simulink model "NN_v01"  (R2018b)
settings: Solver=VariableStepAuto  StartTime=0.0  StopTime=10.0  RelTol=1e-3
values from neighbouring files (symbols this model uses):
  B = 0.5    [Matlab_Newton_simulation_v01.m]    (also in NewtonMethod.m; NewtonMethod_2.m = 0.3; System_parameters.m = 0.3)
  b = f    (= 0.01)    [Matlab_Newton_simulation_v01.m]    (also in NewtonMethod.m; System_parameters.m)
  in_NN_data = [0 -100 -100 -100 -100 -100 -100 -100 -100 -100 -100 -100 ... (160801 elements, 401x401)]    [NN_IO_data.mat]    (also in NN_generate_input_data.m = con2seq(in_NN_data); NN_modelling_v02.m = con2seq(in_NN_data); NN_modelling_v03.m = con2seq(in_NN_data))
  l = 0.1    [Matlab_Newton_simulation_v01.m]    (also in NewtonMethod.m; NewtonMethod_2.m; System_parameters.m)
  m = 0.04    [Matlab_Newton_simulation_v01.m]    (also in NewtonMethod.m = 0.1; NewtonMethod_2.m; System_parameters.m)
  R = 1    [Matlab_Newton_simulation_v01.m]    (also in NewtonMethod.m; NewtonMethod_2.m = 0.1; System_parameters.m = 0.1)
libraries: neural x128
(part 1 of 5)
settings Model: Creator=Tyson  LastModifiedBy=Tyson

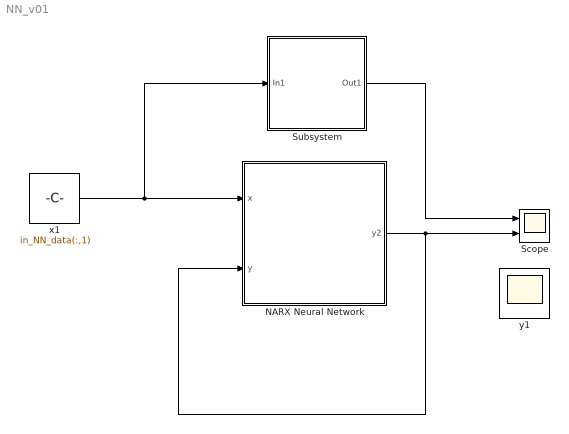
== system NN_v01 ==
  NARX Neural Network : Subsystem  mask{pi_input_1_delayed_1=-1, pi_input_1_delayed_2=-1, pi_input_2_delayed_1=-1, pi_input_2_delayed_2=-1}
      mask prompts: pi_input_1_delayed_1 "Preprocessed initial input 1 state at timestep 0."; pi_input_1_delayed_2 "Preprocessed initial input 1 state at timestep -1."; pi_input_2_delayed_1 "Preprocessed initial input 2 state at timestep 0."; pi_input_2_delayed_2 "Preprocessed initial input 2 state at timestep -1."
      mask help: NARX Neural Network
      mask Display: e = 0.06;c1 = [120 150 230]/255;c2 = ([120 150 230]+0)/383;c3 = ([120 150 230]+128)/383;patch([0 1 1 0],[0 0 1 1],c1);patch([0 1 1 1-e 1-e 0+e],[0 0 1 1-e 0+e 0+e],c2);patch([0 0 1 1-e 0+e 0+e],[0 1 1 1-e 1-e 0+e],c3);plot([0 1 1 0 0],[0 0 1 1 0]);fprintf('NNET');port_label('input',1,' x');port_label('input',2,' y');port_label('output',1,'y2 ');
  Scope : Scope  NumInputPorts=2
  Subsystem : Subsystem
      mask DialogControl Control2 Prompt: BlackBox
  x1 : Constant  Value=in_NN_data(:,1)  SampleTime=-1
      mask Display: e = 0.06;c1 = [120 230 180]/255;c2 = ([120 230 180]+0)/(256+128);c3 = ([120 230 180]+128)/(256+128);patch([0 1 1 0],[0 0 1 1],c1);patch([0 1 1 1-e 1-e 0+e],[0 0 1 1-e 0+e 0+e],c2);patch([0 0 1 1-e 0+e 0+e],[0 1 1 1-e 1-e 0+e],c3);plot([0 1 1 0 0],[0 0 1 1 0]);disp('Constant');
  y1 : Scope
      mask Display: e = 0.06;c1 = [120 230 180]/255;c2 = ([120 230 180]+0)/(256+128);c3 = ([120 230 180]+128)/(256+128);patch([0 1 1 0],[0 0 1 1],c1);patch([0 1 1 1-e 1-e 0+e],[0 0 1 1-e 0+e 0+e],c2);patch([0 0 1 1-e 0+e 0+e],[0 1 1 1-e 1-e 0+e],c3);plot([0 1 1 0 0],[0 0 1 1 0]);plot([0.15 0.85 0.85 0.15 0.15],[0.5 0.5 0.85 0.85 0.5]);
  wires:
  x1/1 -> Subsystem/1(In1), NARX Neural Network/1(x)
  NARX Neural Network/1(y2) -> NARX Neural Network/2(y), Scope/2
  Subsystem/1(Out1) -> Scope/1

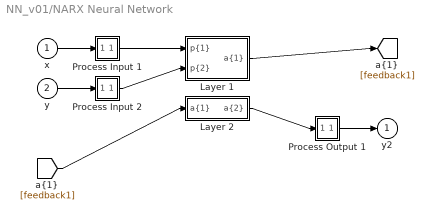
== system NN_v01/NARX Neural Network ==
  x : Inport  PortDimensions=101  SampleTime=1
      mask Display: e = 0.06;c1 = [120 230 180]/255;c2 = ([120 230 180]+0)/(256+128);c3 = ([120 230 180]+128)/(256+128);patch([0 1 1 0],[0 0 1 1],c1);patch([0 1 1 1-e 1-e 0+e],[0 0 1 1-e 0+e 0+e],c2);patch([0 0 1 1-e 0+e 0+e],[0 1 1 1-e 1-e 0+e],c3);plot([0 1 1 0 0],[0 0 1 1 0]);
  y : Inport  Port=2  PortDimensions=101  SampleTime=1
      mask Display: e = 0.06;c1 = [120 230 180]/255;c2 = ([120 230 180]+0)/(256+128);c3 = ([120 230 180]+128)/(256+128);patch([0 1 1 0],[0 0 1 1],c1);patch([0 1 1 1-e 1-e 0+e],[0 0 1 1-e 0+e 0+e],c2);patch([0 0 1 1-e 0+e 0+e],[0 1 1 1-e 1-e 0+e],c3);plot([0 1 1 0 0],[0 0 1 1 0]);
  Layer 1 : Subsystem
      mask Display: e = 0.06;c1 = [120 150 230]/255;c2 = ([120 150 230]+0)/383;c3 = ([120 150 230]+128)/383;patch([0 1 1 0],[0 0 1 1],c1);patch([0 1 1 1-e 1-e 0+e],[0 0 1 1-e 0+e 0+e],c2);patch([0 0 1 1-e 0+e 0+e],[0 1 1 1-e 1-e 0+e],c3);plot([0 1 1 0 0],[0 0 1 1 0]);
  Layer 2 : Subsystem
      mask Display: e = 0.06;c1 = [120 150 230]/255;c2 = ([120 150 230]+0)/383;c3 = ([120 150 230]+128)/383;patch([0 1 1 0],[0 0 1 1],c1);patch([0 1 1 1-e 1-e 0+e],[0 0 1 1-e 0+e 0+e],c2);patch([0 0 1 1-e 0+e 0+e],[0 1 1 1-e 1-e 0+e],c3);plot([0 1 1 0 0],[0 0 1 1 0]);
  Process Input 1 : Subsystem
      mask Display: e = 0.06;c1 = [120 150 230]/255;c2 = ([120 150 230]+0)/383;c3 = ([120 150 230]+128)/383;patch([0 1 1 0],[0 0 1 1],c1);patch([0 1 1 1-e 1-e 0+e],[0 0 1 1-e 0+e 0+e],c2);patch([0 0 1 1-e 0+e 0+e],[0 1 1 1-e 1-e 0+e],c3);plot([0 1 1 0 0],[0 0 1 1 0]);
  Process Input 2 : Subsystem
      mask Display: e = 0.06;c1 = [120 150 230]/255;c2 = ([120 150 230]+0)/383;c3 = ([120 150 230]+128)/383;patch([0 1 1 0],[0 0 1 1],c1);patch([0 1 1 1-e 1-e 0+e],[0 0 1 1-e 0+e 0+e],c2);patch([0 0 1 1-e 0+e 0+e],[0 1 1 1-e 1-e 0+e],c3);plot([0 1 1 0 0],[0 0 1 1 0]);
  Process Output 1 : Subsystem
      mask Display: e = 0.06;c1 = [120 150 230]/255;c2 = ([120 150 230]+0)/383;c3 = ([120 150 230]+128)/383;patch([0 1 1 0],[0 0 1 1],c1);patch([0 1 1 1-e 1-e 0+e],[0 0 1 1-e 0+e 0+e],c2);patch([0 0 1 1-e 0+e 0+e],[0 1 1 1-e 1-e 0+e],c3);plot([0 1 1 0 0],[0 0 1 1 0]);
  y2 : Outport  InitialOutput=[0;0;0;0;0;0;0;0;0;0;0;0;0;0;0;0;0;0;0;0;0;0;0;0;0;0;0;0;0;0;0;0;0;0;0;0;0;0;0;0;0;0;0;0;0;0;0;0;0;0;0;0;0;0;0;0;0;0;0;0;0;0;0;0;0;0;0;0;0;0;0;0;0;0;0;0;0;0;0;0;0;0;0;0;0;0;0;0;0;0;0;0;0;0;0;0;0;0;0;0;0]
      mask Display: e = 0.06;c1 = [120 230 180]/255;c2 = ([120 230 180]+0)/(256+128);c3 = ([120 230 180]+128)/(256+128);patch([0 1 1 0],[0 0 1 1],c1);patch([0 1 1 1-e 1-e 0+e],[0 0 1 1-e 0+e 0+e],c2);patch([0 0 1 1-e 0+e 0+e],[0 1 1 1-e 1-e 0+e],c3);plot([0 1 1 0 0],[0 0 1 1 0]);
  wires:
  x/1 -> Process Input 1/1(x)
  y/1 -> Process Input 2/1(x)
  Process Output 1/1(y) -> y2/1
  Process Input 1/1(p) -> Layer 1/1("p{1}")
  Process Input 2/1(p) -> Layer 1/2("p{2}")
  Layer 1/1("a{1}") -> [feedback1]
  [feedback1] -> Layer 2/1("a{1} ")
  Layer 2/1("a{2}") -> Process Output 1/1(a)

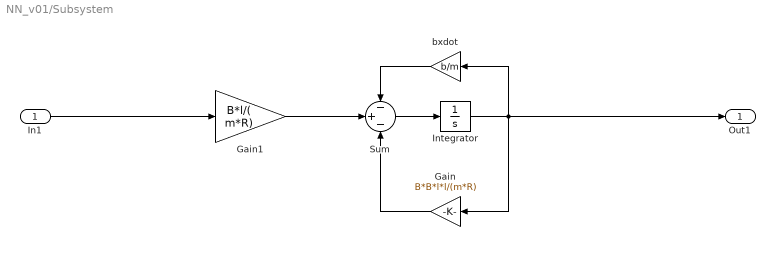
== system NN_v01/Subsystem ==
  In1 : Inport
  Gain : Gain  Gain=B*B*l*l/(m*R)
  Gain1 : Gain  Gain=B*l/( m*R)
  Integrator : Integrator
  Sum : Sum  Inputs=-+-
  bxdot : Gain  Gain=b/m
  Out1 : Outport
  wires:
  Sum/1 -> Integrator/1
  Gain/1 -> Sum/3
  Gain1/1 -> Sum/2
  bxdot/1 -> Sum/1
  Integrator/1 -> Out1/1, bxdot/1, Gain/1
  In1/1 -> Gain1/1

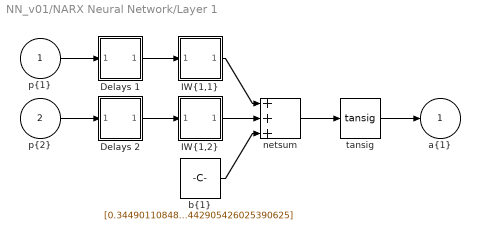
== system NN_v01/NARX Neural Network/Layer 1 ==
  "p{1}" : Inport  PortDimensions=100  SampleTime=1
      mask Display: e = 0.06;c1 = [120 230 180]/255;c2 = ([120 230 180]+0)/(256+128);c3 = ([120 230 180]+128)/(256+128);patch([0 1 1 0],[0 0 1 1],c1);patch([0 1 1 1-e 1-e 0+e],[0 0 1 1-e 0+e 0+e],c2);patch([0 0 1 1-e 0+e 0+e],[0 1 1 1-e 1-e 0+e],c3);plot([0 1 1 0 0],[0 0 1 1 0]);
  "p{2}" : Inport  Port=2  PortDimensions=100  SampleTime=1
      mask Display: e = 0.06;c1 = [120 230 180]/255;c2 = ([120 230 180]+0)/(256+128);c3 = ([120 230 180]+128)/(256+128);patch([0 1 1 0],[0 0 1 1],c1);patch([0 1 1 1-e 1-e 0+e],[0 0 1 1-e 0+e 0+e],c2);patch([0 0 1 1-e 0+e 0+e],[0 1 1 1-e 1-e 0+e],c3);plot([0 1 1 0 0],[0 0 1 1 0]);
  Delays 1 : Subsystem
      mask Display: e = 0.06;c1 = [120 150 230]/255;c2 = ([120 150 230]+0)/383;c3 = ([120 150 230]+128)/383;patch([0 1 1 0],[0 0 1 1],c1);patch([0 1 1 1-e 1-e 0+e],[0 0 1 1-e 0+e 0+e],c2);patch([0 0 1 1-e 0+e 0+e],[0 1 1 1-e 1-e 0+e],c3);plot([0 1 1 0 0],[0 0 1 1 0]);disp('1-2');
  Delays 2 : Subsystem
      mask Display: e = 0.06;c1 = [120 150 230]/255;c2 = ([120 150 230]+0)/383;c3 = ([120 150 230]+128)/383;patch([0 1 1 0],[0 0 1 1],c1);patch([0 1 1 1-e 1-e 0+e],[0 0 1 1-e 0+e 0+e],c2);patch([0 0 1 1-e 0+e 0+e],[0 1 1 1-e 1-e 0+e],c3);plot([0 1 1 0 0],[0 0 1 1 0]);disp('1-2');
  "IW{1,1}" : Subsystem
      mask Display: e = 0.06;c1 = [120 150 230]/255;c2 = ([120 150 230]+0)/383;c3 = ([120 150 230]+128)/383;patch([0 1 1 0],[0 0 1 1],c1);patch([0 1 1 1-e 1-e 0+e],[0 0 1 1-e 0+e 0+e],c2);patch([0 0 1 1-e 0+e 0+e],[0 1 1 1-e 1-e 0+e],c3);plot([0 1 1 0 0],[0 0 1 1 0]);disp('W');
  "IW{1,2}" : Subsystem
      mask Display: e = 0.06;c1 = [120 150 230]/255;c2 = ([120 150 230]+0)/383;c3 = ([120 150 230]+128)/383;patch([0 1 1 0],[0 0 1 1],c1);patch([0 1 1 1-e 1-e 0+e],[0 0 1 1-e 0+e 0+e],c2);patch([0 0 1 1-e 0+e 0+e],[0 1 1 1-e 1-e 0+e],c3);plot([0 1 1 0 0],[0 0 1 1 0]);disp('W');
  "b{1}" : Constant  Value=[0.34490110848554278444311194107285700738430023193359375;-0.55926377926860249001350666731013916432857513427734375;0.08828364470528819729633340784857864491641521453857421875;0.47063354920653821533704785906593315303325653076171875;0.0163244137557161834994889915151361492462456226348876953125;0.380666321851039490820056698794360272586345672607421875;0.473534513113422317331924205063842236995697021484375;0.0303941138129983599858174869723370647989213466644287109375;-0.00010565009611801054359263296600346393461222760379314422607421875;-0.0342241349195050725828792792526655830442905426025390625]
      mask Display: e = 0.06;c1 = [120 150 230]/255;c2 = ([120 150 230]+0)/383;c3 = ([120 150 230]+128)/383;patch([0 1 1 0],[0 0 1 1],c1);patch([0 1 1 1-e 1-e 0+e],[0 0 1 1-e 0+e 0+e],c2);patch([0 0 1 1-e 0+e 0+e],[0 1 1 1-e 1-e 0+e],c3);plot([0 1 1 0 0],[0 0 1 1 0]);disp('b');
  netsum : Sum  Inputs=3  SaturateOnIntegerOverflow=on  InputSameDT=on  OutDataTypeStr=Inherit: Same as first input
      mask Display: e = 0.06;c1 = [120 150 230]/255;c2 = ([120 150 230]+0)/383;c3 = ([120 150 230]+128)/383;patch([0 1 1 0],[0 0 1 1],c1);patch([0 1 1 1-e 1-e 0+e],[0 0 1 1-e 0+e 0+e],c2);patch([0 0 1 1-e 0+e 0+e],[0 1 1 1-e 1-e 0+e],c3);plot([0 1 1 0 0],[0 0 1 1 0]);disp('+');
  tansig : neural/Transfer Functions/tansig
  "a{1}" : Outport  InitialOutput=[0;0;0;0;0;0;0;0;0;0]
      mask Display: e = 0.06;c1 = [120 230 180]/255;c2 = ([120 230 180]+0)/(256+128);c3 = ([120 230 180]+128)/(256+128);patch([0 1 1 0],[0 0 1 1],c1);patch([0 1 1 1-e 1-e 0+e],[0 0 1 1-e 0+e 0+e],c2);patch([0 0 1 1-e 0+e 0+e],[0 1 1 1-e 1-e 0+e],c3);plot([0 1 1 0 0],[0 0 1 1 0]);
  wires:
  "p{1}"/1 -> Delays 1/1("p{1}")
  Delays 1/1("pd{1,1}") -> "IW{1,1}"/1("pd{1,1}")
  "IW{1,1}"/1("iz{1,1}") -> netsum/1
  "p{2}"/1 -> Delays 2/1("p{1}")
  Delays 2/1("pd{1,2}") -> "IW{1,2}"/1("pd{1,2}")
  "IW{1,2}"/1("iz{1,2}") -> netsum/2
  "b{1}"/1 -> netsum/3
  netsum/1 -> tansig/1
  tansig/1 -> "a{1}"/1

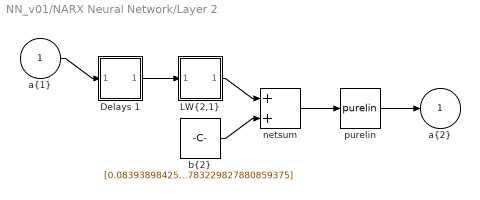
== system NN_v01/NARX Neural Network/Layer 2 ==
  "a{1} " : Inport  PortDimensions=10  SampleTime=1
      mask Display: e = 0.06;c1 = [120 230 180]/255;c2 = ([120 230 180]+0)/(256+128);c3 = ([120 230 180]+128)/(256+128);patch([0 1 1 0],[0 0 1 1],c1);patch([0 1 1 1-e 1-e 0+e],[0 0 1 1-e 0+e 0+e],c2);patch([0 0 1 1-e 0+e 0+e],[0 1 1 1-e 1-e 0+e],c3);plot([0 1 1 0 0],[0 0 1 1 0]);
  Delays 1 : Subsystem
      mask Display: e = 0.06;c1 = [120 150 230]/255;c2 = ([120 150 230]+0)/383;c3 = ([120 150 230]+128)/383;patch([0 1 1 0],[0 0 1 1],c1);patch([0 1 1 1-e 1-e 0+e],[0 0 1 1-e 0+e 0+e],c2);patch([0 0 1 1-e 0+e 0+e],[0 1 1 1-e 1-e 0+e],c3);plot([0 1 1 0 0],[0 0 1 1 0]);disp('0');
  "LW{2,1}" : Subsystem
      mask Display: e = 0.06;c1 = [120 150 230]/255;c2 = ([120 150 230]+0)/383;c3 = ([120 150 230]+128)/383;patch([0 1 1 0],[0 0 1 1],c1);patch([0 1 1 1-e 1-e 0+e],[0 0 1 1-e 0+e 0+e],c2);patch([0 0 1 1-e 0+e 0+e],[0 1 1 1-e 1-e 0+e],c3);plot([0 1 1 0 0],[0 0 1 1 0]);disp('W');
  "b{2}" : Constant  Value=[0.08393898425384989370190425006512668915092945098876953125;0.04747955954920869692248430737890885211527347564697265625;0.02259412956298940955424114918059785850346088409423828125;0.0189850525832074117082992614768954808823764324188232421875;-0.021115224393390634449740872469192254357039928436279296875;-0.0258363266266243007951430854518548585474491119384765625;-0.032480391177460994633907631623515044339001178741455078125;-0.00530185149898763398434997640151777886785566806793212890625;0.00082595733270498269788795209223053461755625903606414794921875;0.00153775931011657248335955383566897580749355256557464599609375;-0.020679742413263597911043945032361079938709735870361328125;-0.0177142011664902405965182907721100491471588611602783203125;-0.032660583320958509745413067548724939115345478057861328125;-0.03167603138593400036171487954561598598957061767578125;-0.02560287967276560217033676281062071211636066436767578125;-0.01468973685666209900990697434508547303266823291778564453125;-0.0287572723231526994336348934666602872312068939208984375;-0.01438192548970657937135175785670071491040289402008056640625;-0.01225306330625217966778794931315132998861372470855712890625;-0.009015829424581602025146054302240372635424137115478515625;-0.0224190206360676824726141376231680624186992645263671875;-0.0162041639024568494276135055542908958159387111663818359375;0.00463628568182163254551841902184605714865028858184814453125;-0.017249539041738481959242790253483690321445465087890625;-0.0093907194819392129925272882928766193799674510955810546875;0.00103156476558706466928327927234931848943233489990234375;-0.0149805915005030397535445985113256028853356838226318359375;-0.0117658372520909083880358281248845742084085941314697265625;-0.002292463185382479125273835762754970346577465534210205078125;-0.0115253284335917853542508026976065593771636486053466796875;-0.000676344485529874715756815106715293950401246547698974609375;-0.0211093999094044103281841984198763384483754634857177734375;-0.0033268637067907619840612110095889875083230435848236083984375;-0.0277640599743354289652419453204856836237013339996337890625;0.00410158032873014603836292479854819248430430889129638671875;-0.019817410413248894018867218846935429610311985015869140625;-0.03181619165364106549542810853381524793803691864013671875;-0.005128465510424081059970280449533674982376396656036376953125;-0.0122950128646857233249978236244714935310184955596923828125;-0.0296459773916183007280711336761669372208416461944580078125;-0.02841264500203134757416734146318049170076847076416015625;-0.0288484832263984948552693055034978897310793399810791015625;-0.0316585468321592122808993963190005160868167877197265625;-0.01425623173418808474488539417279753251932561397552490234375;-0.0326474212064222502061028308162349276244640350341796875;-0.026458854464259225214295412342835334129631519317626953125;-0.041621208256695275962133706570966751314699649810791015625;-0.0323289680718874539167018156149424612522125244140625;-0.0148329882382925264117101704641754622571170330047607421875;-0.01090351148061602555572324746435697306878864765167236328125;-0.038850136436738465228746264301662449724972248077392578125;-0.03859829631133258887043524509863345883786678314208984375;-0.006839581773198071500130534872141652158461511135101318359375;-0.0259010284650814902318582966245230636559426784515380859375;-0.03254737113984364216268119207597919739782810211181640625;-0.02189820350106060076189606888874550350010395050048828125;-0.005298122488479149218287833633667105459608137607574462890625;-0.020306466616356773358109677474203635938465595245361328125;-0.03097649086438274135257842090140911750495433807373046875;-0.0365192638172040784372285315839690156280994415283203125;-0.0156068747337300868516241081351836328394711017608642578125;-0.0275454361412660712893352155106185819022357463836669921875;-0.029019398236701375581869655206901370547711849212646484375;-0.030534494348092237892000611054754699580371379852294921875;-0.0122323399612508480760464379955010372214019298553466796875 ...(+2140 chars)]
      mask Display: e = 0.06;c1 = [120 150 230]/255;c2 = ([120 150 230]+0)/383;c3 = ([120 150 230]+128)/383;patch([0 1 1 0],[0 0 1 1],c1);patch([0 1 1 1-e 1-e 0+e],[0 0 1 1-e 0+e 0+e],c2);patch([0 0 1 1-e 0+e 0+e],[0 1 1 1-e 1-e 0+e],c3);plot([0 1 1 0 0],[0 0 1 1 0]);disp('b');
  netsum : Sum  Inputs=2  SaturateOnIntegerOverflow=on  InputSameDT=on  OutDataTypeStr=Inherit: Same as first input
      mask Display: e = 0.06;c1 = [120 150 230]/255;c2 = ([120 150 230]+0)/383;c3 = ([120 150 230]+128)/383;patch([0 1 1 0],[0 0 1 1],c1);patch([0 1 1 1-e 1-e 0+e],[0 0 1 1-e 0+e 0+e],c2);patch([0 0 1 1-e 0+e 0+e],[0 1 1 1-e 1-e 0+e],c3);plot([0 1 1 0 0],[0 0 1 1 0]);disp('+');
  purelin : neural/Transfer Functions/purelin
  "a{2}" : Outport  InitialOutput=[0;0;0;0;0;0;0;0;0;0;0;0;0;0;0;0;0;0;0;0;0;0;0;0;0;0;0;0;0;0;0;0;0;0;0;0;0;0;0;0;0;0;0;0;0;0;0;0;0;0;0;0;0;0;0;0;0;0;0;0;0;0;0;0;0;0;0;0;0;0;0;0;0;0;0;0;0;0;0;0;0;0;0;0;0;0;0;0;0;0;0;0;0;0;0;0;0;0;0;0]
      mask Display: e = 0.06;c1 = [120 230 180]/255;c2 = ([120 230 180]+0)/(256+128);c3 = ([120 230 180]+128)/(256+128);patch([0 1 1 0],[0 0 1 1],c1);patch([0 1 1 1-e 1-e 0+e],[0 0 1 1-e 0+e 0+e],c2);patch([0 0 1 1-e 0+e 0+e],[0 1 1 1-e 1-e 0+e],c3);plot([0 1 1 0 0],[0 0 1 1 0]);
  wires:
  "a{1} "/1 -> Delays 1/1("p{2}")
  Delays 1/1("pd{2,1}") -> "LW{2,1}"/1("ad{2,1}")
  "LW{2,1}"/1("lz{2,1}") -> netsum/1
  "b{2}"/1 -> netsum/2
  netsum/1 -> purelin/1
  purelin/1 -> "a{2}"/1

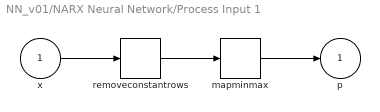
== system NN_v01/NARX Neural Network/Process Input 1 ==
  x : Inport  PortDimensions=101  SampleTime=1
      mask Display: e = 0.06;c1 = [120 230 180]/255;c2 = ([120 230 180]+0)/(256+128);c3 = ([120 230 180]+128)/(256+128);patch([0 1 1 0],[0 0 1 1],c1);patch([0 1 1 1-e 1-e 0+e],[0 0 1 1-e 0+e 0+e],c2);patch([0 0 1 1-e 0+e 0+e],[0 1 1 1-e 1-e 0+e],c3);plot([0 1 1 0 0],[0 0 1 1 0]);
  mapminmax : neural/Processing Functions/mapminmax  xmin=[-50;-50;-50;-50;-50;-50;-50;-50;-50;-50;-50;-50;-50;-50;-50;-50;-50;-50;-50;-50;-50;-50;-50;-50;-50;-50;-50;-50;-50;-50;-50;-50;-50;-50;-50;-50;-50;-50;-50;-50;-50;-50;-50;-50;-50;-50;-50;-50;-50;-50;-50;-50;-50;-50;-50;-50;-50;-50;-50;-50;-50;-50;-50;-50;-50;-50;-50;-50;-50;-50;-50;-50;-50;-50;-50;-50;-50;-50;-50;-50;-50;-50;-50;-50;-50;-50;-50;-50;-50;-50;-50;-50;-50;-50;-50;-50;-50;-50;-50;-50]  xmax=[50;50;50;50;50;50;50;50;50;50;50;50;50;50;50;50;50;50;50;50;50;50;50;50;50;50;50;50;50;50;50;50;50;50;50;50;50;50;50;50;50;50;50;50;50;50;50;50;50;50;50;50;50;50;50;50;50;50;50;50;50;50;50;50;50;50;50;50;50;50;50;50;50;50;50;50;50;50;50;50;50;50;50;50;50;50;50;50;50;50;50;50;50;50;50;50;50;50;50;50]  ymin=-1  ymax=1
  removeconstantrows : neural/Processing Functions/removeconstantrows  inputSize=101  keep=[2 3 4 5 6 7 8 9 10 11 12 13 14 15 16 17 18 19 20 21 22 23 24 25 26 27 28 29 30 31 32 33 34 35 36 37 38 39 40 41 42 43 44 45 46 47 48 49 50 51 52 53 54 55 56 57 58 59 60 61 62 63 64 65 66 67 68 69 70 71 72 73 74 75 76 77 78 79 80 81 82 83 84 85 86 87 88 89 90 91 92 93 94 95 96 97 98 99 100 101]
      settings: SourceProductName=Neural Network Toolbox  SourceProductBaseCode=NN
  p : Outport  PortDimensions=100  SampleTime=1
      mask Display: e = 0.06;c1 = [120 230 180]/255;c2 = ([120 230 180]+0)/(256+128);c3 = ([120 230 180]+128)/(256+128);patch([0 1 1 0],[0 0 1 1],c1);patch([0 1 1 1-e 1-e 0+e],[0 0 1 1-e 0+e 0+e],c2);patch([0 0 1 1-e 0+e 0+e],[0 1 1 1-e 1-e 0+e],c3);plot([0 1 1 0 0],[0 0 1 1 0]);
  wires:
  x/1 -> removeconstantrows/1
  removeconstantrows/1 -> mapminmax/1
  mapminmax/1 -> p/1

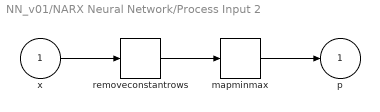
== system NN_v01/NARX Neural Network/Process Input 2 ==
  x : Inport  PortDimensions=101  SampleTime=1
      mask Display: e = 0.06;c1 = [120 230 180]/255;c2 = ([120 230 180]+0)/(256+128);c3 = ([120 230 180]+128)/(256+128);patch([0 1 1 0],[0 0 1 1],c1);patch([0 1 1 1-e 1-e 0+e],[0 0 1 1-e 0+e 0+e],c2);patch([0 0 1 1-e 0+e 0+e],[0 1 1 1-e 1-e 0+e],c3);plot([0 1 1 0 0],[0 0 1 1 0]);
  mapminmax : neural/Processing Functions/mapminmax  xmin=[-18.453125;-54.2205659473063121822633547708;-88.3287647166492035921692149714;-120.854693116249151785268622916;-151.871752252388432680163532495;-181.449938173334970770156360231;-209.655999829087903663094039075;-236.553589703412313838271074928;-262.203407458093295190337812528;-286.663336913571072273043682799;-309.988576675080253153282683343;-332.231764699077018576645059511;-353.443097081062433062470518053;-373.670441332869870620925212279;-392.95944440504888461873633787;-411.353635698119205699185840786;-428.894525295159496636188123375;-445.621697637412523818056797609;-461.572900854303213691309792921;-476.784131949461141175561351702;-491.289718034985355643584625795;-505.122393797273446125473128632;-518.313375369230925571173429489;-530.892430775568186618329491466;-542.88794711015907523687928915;-554.326994597059069747047033161;-565.235387679749578637711238116;-575.637743276468654585187323391;-585.557536333092230051988735795;-595.017152798931306278973352164;-604.037940144996241542685311288;-612.640255538732276363589335233;-620.843511783941039539058692753;-628.666221129561904490401502699;-636.126037046174928946129512042;-643.239794064503257686737924814;-650.023545765817630126548465341;-656.49260100997605604788986966;-662.661558482854275098361540586;-668.544339641130022755532991141;-674.154220128767292408156208694;-679.503859736098547728033736348;-684.605330969112401362508535385;-689.470146293419929861556738615;-694.109284114380670871469192207;-698.533213552016832181834615767;-702.75191806662667204363970086;-706.77491798841094805538887158;-710.611292001956485364644322544;-714.269697634059980373422149569;-717.758390791126998919935431331;-721.085244390236653089232277125;-724.257766125915509292099159211;-727.283115412715460479375906289;-730.168119541830719754216261208;-732.919289088212508431752212346;-735.542832602952557863318361342;-738.044670624090372257342096418;-740.430449037463176864548586309;-742.705551817748983012279495597;-744.875113178456786044989712536;-746.94402915828118239005561918;-748.916968669969492111704312265;-750.798384036634843141655437648;-752.592521039292023488087579608;-754.30342849829128226701868698;-755.934967410271951848699245602;-757.490819661254477068723645061;-758.974496335535491198243107647;-760.389345639134489829302765429;-761.738560455674360127886757255;-763.025185551746631062997039407;-764.252124448021277203224599361;-765.42214597160818811971694231;-766.537890504455958762264344841;-767.601875941889034038467798382;-768.61650337472985938802594319;-769.584062507829344212950672954;-770.506736827232543873833492398;-771.386608527641215005132835358;-772.225663211292498999682720751;-773.025794368858100824581924826;-773.788807652475384202261921018;-774.516424950554096540145110339;-775.210288273553373983304481953;-775.871963459499283999321050942;-776.502943707603549228224437684;-777.104652947959152697876561433;-777.678449054916768545808736235;-778.225626911392964757396839559;-778.74742133102631669316906482;-779.245009844775722740450873971;-779.719515358248486336378846318;-780.17200868575605454680044204;-780.603510966815747451619245112;-781.014995970551126447389833629;-781.407392293192401666601654142;-781.781585453634647819853853434;-782.13841989178467883903067559;-782.478700874203809689788613468]  xmax=[18.453125;54.2205659473063121822633547708;88.3287647166492035921692149714;120.854693116249151785268622916;151.871752252388432680163532495;181.449938173334970770156360231;209.655999829087903663094039075;236.553589703412313838271074928;262.203407458093295190337812528;286.663336913571072273043682799;309.988576675080253153282683343;332.231764699077018576645059511;353.443097081062433062470518053;373.670441332869870620925212279;392.95944440504888461873633787;411.353635698119205699185840786;428.894525295159496636188123375;445.621697637412523818056797609;461.572900854303213691309792921;476.784131949461141175561351702;491.289718034985355643584625795;505.122393797273446125473128632;518.313375369230925571173429489;530.892430775568186618329491466;542.88794711015907523687928915;554.326994597059069747047033161;565.235387679749578637711238116;575.637743276468654585187323391;585.557536333092230051988735795;595.017152798931306278973352164;604.037940144996241542685311288;612.640255538732276363589335233;620.843511783941039539058692753;628.666221129561904490401502699;636.126037046174928946129512042;643.239794064503257686737924814;650.023545765817630126548465341;656.49260100997605604788986966;662.661558482854275098361540586;668.544339641130022755532991141;674.154220128767292408156208694;679.503859736098547728033736348;684.605330969112401362508535385;689.470146293419929861556738615;694.109284114380670871469192207;698.533213552016832181834615767;702.75191806662667204363970086;706.77491798841094805538887158;710.611292001956485364644322544;714.269697634059980373422149569;717.758390791126998919935431331;721.085244390236653089232277125;724.257766125915509292099159211;727.283115412715460479375906289;730.168119541830719754216261208;732.919289088212508431752212346;735.542832602952557863318361342;738.044670624090372257342096418;740.430449037463176864548586309;742.705551817748983012279495597;744.875113178456786044989712536;746.94402915828118239005561918;748.916968669969492111704312265;750.798384036634843141655437648;752.592521039292023488087579608;754.30342849829128226701868698;755.934967410271951848699245602;757.490819661254477068723645061;758.974496335535491198243107647;760.389345639134489829302765429;761.738560455674360127886757255;763.025185551746631062997039407;764.252124448021277203224599361;765.42214597160818811971694231;766.537890504455958762264344841;767.601875941889034038467798382;768.61650337472985938802594319;769.584062507829344212950672954;770.506736827232543873833492398;771.386608527641215005132835358;772.225663211292498999682720751;773.025794368858100824581924826;773.788807652475384202261921018;774.516424950554096540145110339;775.210288273553373983304481953;775.871963459499283999321050942;776.502943707603549228224437684;777.104652947959152697876561433;777.678449054916768545808736235;778.225626911392964757396839559;778.74742133102631669316906482;779.245009844775722740450873971;779.719515358248486336378846318;780.17200868575605454680044204;780.603510966815747451619245112;781.014995970551126447389833629;781.407392293192401666601654142;781.781585453634647819853853434;782.13841989178467883903067559;782.478700874203809689788613468]  ymin=-1  ymax=1
  removeconstantrows : neural/Processing Functions/removeconstantrows  inputSize=101  keep=[2 3 4 5 6 7 8 9 10 11 12 13 14 15 16 17 18 19 20 21 22 23 24 25 26 27 28 29 30 31 32 33 34 35 36 37 38 39 40 41 42 43 44 45 46 47 48 49 50 51 52 53 54 55 56 57 58 59 60 61 62 63 64 65 66 67 68 69 70 71 72 73 74 75 76 77 78 79 80 81 82 83 84 85 86 87 88 89 90 91 92 93 94 95 96 97 98 99 100 101]
      settings: SourceProductName=Neural Network Toolbox  SourceProductBaseCode=NN
  p : Outport  PortDimensions=100  SampleTime=1
      mask Display: e = 0.06;c1 = [120 230 180]/255;c2 = ([120 230 180]+0)/(256+128);c3 = ([120 230 180]+128)/(256+128);patch([0 1 1 0],[0 0 1 1],c1);patch([0 1 1 1-e 1-e 0+e],[0 0 1 1-e 0+e 0+e],c2);patch([0 0 1 1-e 0+e 0+e],[0 1 1 1-e 1-e 0+e],c3);plot([0 1 1 0 0],[0 0 1 1 0]);
  wires:
  x/1 -> removeconstantrows/1
  removeconstantrows/1 -> mapminmax/1
  mapminmax/1 -> p/1

== system NN_v01/NARX Neural Network/Process Output 1 ==
  a : Inport  PortDimensions=100  SampleTime=1
      mask Display: e = 0.06;c1 = [120 230 180]/255;c2 = ([120 230 180]+0)/(256+128);c3 = ([120 230 180]+128)/(256+128);patch([0 1 1 0],[0 0 1 1],c1);patch([0 1 1 1-e 1-e 0+e],[0 0 1 1-e 0+e 0+e],c2);patch([0 0 1 1-e 0+e 0+e],[0 1 1 1-e 1-e 0+e],c3);plot([0 1 1 0 0],[0 0 1 1 0]);
  mapminmax_reverse : neural/Processing Functions/mapminmax_reverse  xmin=[-18.453125;-54.2205659473063121822633547708;-88.3287647166492035921692149714;-120.854693116249151785268622916;-151.871752252388432680163532495;-181.449938173334970770156360231;-209.655999829087903663094039075;-236.553589703412313838271074928;-262.203407458093295190337812528;-286.663336913571072273043682799;-309.988576675080253153282683343;-332.231764699077018576645059511;-353.443097081062433062470518053;-373.670441332869870620925212279;-392.95944440504888461873633787;-411.353635698119205699185840786;-428.894525295159496636188123375;-445.621697637412523818056797609;-461.572900854303213691309792921;-476.784131949461141175561351702;-491.289718034985355643584625795;-505.122393797273446125473128632;-518.313375369230925571173429489;-530.892430775568186618329491466;-542.88794711015907523687928915;-554.326994597059069747047033161;-565.235387679749578637711238116;-575.637743276468654585187323391;-585.557536333092230051988735795;-595.017152798931306278973352164;-604.037940144996241542685311288;-612.640255538732276363589335233;-620.843511783941039539058692753;-628.666221129561904490401502699;-636.126037046174928946129512042;-643.239794064503257686737924814;-650.023545765817630126548465341;-656.49260100997605604788986966;-662.661558482854275098361540586;-668.544339641130022755532991141;-674.154220128767292408156208694;-679.503859736098547728033736348;-684.605330969112401362508535385;-689.470146293419929861556738615;-694.109284114380670871469192207;-698.533213552016832181834615767;-702.75191806662667204363970086;-706.77491798841094805538887158;-710.611292001956485364644322544;-714.269697634059980373422149569;-717.758390791126998919935431331;-721.085244390236653089232277125;-724.257766125915509292099159211;-727.283115412715460479375906289;-730.168119541830719754216261208;-732.919289088212508431752212346;-735.542832602952557863318361342;-738.044670624090372257342096418;-740.430449037463176864548586309;-742.705551817748983012279495597;-744.875113178456786044989712536;-746.94402915828118239005561918;-748.916968669969492111704312265;-750.798384036634843141655437648;-752.592521039292023488087579608;-754.30342849829128226701868698;-755.934967410271951848699245602;-757.490819661254477068723645061;-758.974496335535491198243107647;-760.389345639134489829302765429;-761.738560455674360127886757255;-763.025185551746631062997039407;-764.252124448021277203224599361;-765.42214597160818811971694231;-766.537890504455958762264344841;-767.601875941889034038467798382;-768.61650337472985938802594319;-769.584062507829344212950672954;-770.506736827232543873833492398;-771.386608527641215005132835358;-772.225663211292498999682720751;-773.025794368858100824581924826;-773.788807652475384202261921018;-774.516424950554096540145110339;-775.210288273553373983304481953;-775.871963459499283999321050942;-776.502943707603549228224437684;-777.104652947959152697876561433;-777.678449054916768545808736235;-778.225626911392964757396839559;-778.74742133102631669316906482;-779.245009844775722740450873971;-779.719515358248486336378846318;-780.17200868575605454680044204;-780.603510966815747451619245112;-781.014995970551126447389833629;-781.407392293192401666601654142;-781.781585453634647819853853434;-782.13841989178467883903067559;-782.478700874203809689788613468]  xmax=[18.453125;54.2205659473063121822633547708;88.3287647166492035921692149714;120.854693116249151785268622916;151.871752252388432680163532495;181.449938173334970770156360231;209.655999829087903663094039075;236.553589703412313838271074928;262.203407458093295190337812528;286.663336913571072273043682799;309.988576675080253153282683343;332.231764699077018576645059511;353.443097081062433062470518053;373.670441332869870620925212279;392.95944440504888461873633787;411.353635698119205699185840786;428.894525295159496636188123375;445.621697637412523818056797609;461.572900854303213691309792921;476.784131949461141175561351702;491.289718034985355643584625795;505.122393797273446125473128632;518.313375369230925571173429489;530.892430775568186618329491466;542.88794711015907523687928915;554.326994597059069747047033161;565.235387679749578637711238116;575.637743276468654585187323391;585.557536333092230051988735795;595.017152798931306278973352164;604.037940144996241542685311288;612.640255538732276363589335233;620.843511783941039539058692753;628.666221129561904490401502699;636.126037046174928946129512042;643.239794064503257686737924814;650.023545765817630126548465341;656.49260100997605604788986966;662.661558482854275098361540586;668.544339641130022755532991141;674.154220128767292408156208694;679.503859736098547728033736348;684.605330969112401362508535385;689.470146293419929861556738615;694.109284114380670871469192207;698.533213552016832181834615767;702.75191806662667204363970086;706.77491798841094805538887158;710.611292001956485364644322544;714.269697634059980373422149569;717.758390791126998919935431331;721.085244390236653089232277125;724.257766125915509292099159211;727.283115412715460479375906289;730.168119541830719754216261208;732.919289088212508431752212346;735.542832602952557863318361342;738.044670624090372257342096418;740.430449037463176864548586309;742.705551817748983012279495597;744.875113178456786044989712536;746.94402915828118239005561918;748.916968669969492111704312265;750.798384036634843141655437648;752.592521039292023488087579608;754.30342849829128226701868698;755.934967410271951848699245602;757.490819661254477068723645061;758.974496335535491198243107647;760.389345639134489829302765429;761.738560455674360127886757255;763.025185551746631062997039407;764.252124448021277203224599361;765.42214597160818811971694231;766.537890504455958762264344841;767.601875941889034038467798382;768.61650337472985938802594319;769.584062507829344212950672954;770.506736827232543873833492398;771.386608527641215005132835358;772.225663211292498999682720751;773.025794368858100824581924826;773.788807652475384202261921018;774.516424950554096540145110339;775.210288273553373983304481953;775.871963459499283999321050942;776.502943707603549228224437684;777.104652947959152697876561433;777.678449054916768545808736235;778.225626911392964757396839559;778.74742133102631669316906482;779.245009844775722740450873971;779.719515358248486336378846318;780.17200868575605454680044204;780.603510966815747451619245112;781.014995970551126447389833629;781.407392293192401666601654142;781.781585453634647819853853434;782.13841989178467883903067559;782.478700874203809689788613468]  ymin=-1  ymax=1
  removeconstantrows_reverse : neural/Processing Functions/removeconstantrows_reverse  inputSize=101  constants=0  rearrange=[101 1 2 3 4 5 6 7 8 9 10 11 12 13 14 15 16 17 18 19 20 21 22 23 24 25 26 27 28 29 30 31 32 33 34 35 36 37 38 39 40 41 42 43 44 45 46 47 48 49 50 51 52 53 54 55 56 57 58 59 60 61 62 63 64 65 66 67 68 69 70 71 72 73 74 75 76 77 78 79 80 81 82 83 84 85 86 87 88 89 90 91 92 93 94 95 96 97 98 99 100]
      settings: SourceProductName=Neural Network Toolbox  SourceProductBaseCode=NN
  y : Outport  PortDimensions=101  SampleTime=1
      mask Display: e = 0.06;c1 = [120 230 180]/255;c2 = ([120 230 180]+0)/(256+128);c3 = ([120 230 180]+128)/(256+128);patch([0 1 1 0],[0 0 1 1],c1);patch([0 1 1 1-e 1-e 0+e],[0 0 1 1-e 0+e 0+e],c2);patch([0 0 1 1-e 0+e 0+e],[0 1 1 1-e 1-e 0+e],c3);plot([0 1 1 0 0],[0 0 1 1 0]);
  wires:
  a/1 -> mapminmax_reverse/1
  mapminmax_reverse/1 -> removeconstantrows_reverse/1
  removeconstantrows_reverse/1 -> y/1

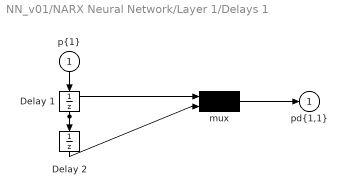
== system NN_v01/NARX Neural Network/Layer 1/Delays 1 ==
  "p{1}" : Inport  PortDimensions=100  SampleTime=1
      mask Display: e = 0.06;c1 = [120 230 180]/255;c2 = ([120 230 180]+0)/(256+128);c3 = ([120 230 180]+128)/(256+128);patch([0 1 1 0],[0 0 1 1],c1);patch([0 1 1 1-e 1-e 0+e],[0 0 1 1-e 0+e 0+e],c2);patch([0 0 1 1-e 0+e 0+e],[0 1 1 1-e 1-e 0+e],c3);plot([0 1 1 0 0],[0 0 1 1 0]);
  Delay 1 : UnitDelay  InitialCondition=pi_input_1_delayed_1
      mask Display: e = 0.06;c1 = [120 150 230]/255;c2 = ([120 150 230]+0)/383;c3 = ([120 150 230]+128)/383;patch([0 1 1 0],[0 0 1 1],c1);patch([0 1 1 1-e 1-e 0+e],[0 0 1 1-e 0+e 0+e],c2);patch([0 0 1 1-e 0+e 0+e],[0 1 1 1-e 1-e 0+e],c3);plot([0 1 1 0 0],[0 0 1 1 0]);disp('D')
  Delay 2 : UnitDelay  InitialCondition=pi_input_1_delayed_2
      mask Display: e = 0.06;c1 = [120 150 230]/255;c2 = ([120 150 230]+0)/383;c3 = ([120 150 230]+128)/383;patch([0 1 1 0],[0 0 1 1],c1);patch([0 1 1 1-e 1-e 0+e],[0 0 1 1-e 0+e 0+e],c2);patch([0 0 1 1-e 0+e 0+e],[0 1 1 1-e 1-e 0+e],c3);plot([0 1 1 0 0],[0 0 1 1 0]);disp('D')
  mux : Mux  Inputs=2
      mask Display: e = 0.06;c1 = [120 150 230]/255;c2 = ([120 150 230]+0)/383;c3 = ([120 150 230]+128)/383;patch([0 1 1 0],[0 0 1 1],c1);patch([0 1 1 1-e 1-e 0+e],[0 0 1 1-e 0+e 0+e],c2);patch([0 0 1 1-e 0+e 0+e],[0 1 1 1-e 1-e 0+e],c3);plot([0 1 1 0 0],[0 0 1 1 0]);disp('Mux')
  "pd{1,1}" : Outport
      mask Display: e = 0.06;c1 = [120 230 180]/255;c2 = ([120 230 180]+0)/(256+128);c3 = ([120 230 180]+128)/(256+128);patch([0 1 1 0],[0 0 1 1],c1);patch([0 1 1 1-e 1-e 0+e],[0 0 1 1-e 0+e 0+e],c2);patch([0 0 1 1-e 0+e 0+e],[0 1 1 1-e 1-e 0+e],c3);plot([0 1 1 0 0],[0 0 1 1 0]);
  wires:
  "p{1}"/1 -> Delay 1/1
  Delay 1/1 -> Delay 2/1, mux/1
  Delay 2/1 -> mux/2
  mux/1 -> "pd{1,1}"/1

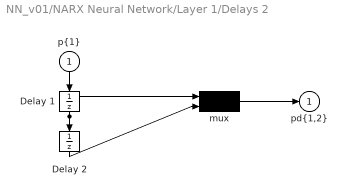
== system NN_v01/NARX Neural Network/Layer 1/Delays 2 ==
  "p{1}" : Inport  PortDimensions=100  SampleTime=1
      mask Display: e = 0.06;c1 = [120 230 180]/255;c2 = ([120 230 180]+0)/(256+128);c3 = ([120 230 180]+128)/(256+128);patch([0 1 1 0],[0 0 1 1],c1);patch([0 1 1 1-e 1-e 0+e],[0 0 1 1-e 0+e 0+e],c2);patch([0 0 1 1-e 0+e 0+e],[0 1 1 1-e 1-e 0+e],c3);plot([0 1 1 0 0],[0 0 1 1 0]);
  Delay 1 : UnitDelay  InitialCondition=pi_input_2_delayed_1
      mask Display: e = 0.06;c1 = [120 150 230]/255;c2 = ([120 150 230]+0)/383;c3 = ([120 150 230]+128)/383;patch([0 1 1 0],[0 0 1 1],c1);patch([0 1 1 1-e 1-e 0+e],[0 0 1 1-e 0+e 0+e],c2);patch([0 0 1 1-e 0+e 0+e],[0 1 1 1-e 1-e 0+e],c3);plot([0 1 1 0 0],[0 0 1 1 0]);disp('D')
  Delay 2 : UnitDelay  InitialCondition=pi_input_2_delayed_2
      mask Display: e = 0.06;c1 = [120 150 230]/255;c2 = ([120 150 230]+0)/383;c3 = ([120 150 230]+128)/383;patch([0 1 1 0],[0 0 1 1],c1);patch([0 1 1 1-e 1-e 0+e],[0 0 1 1-e 0+e 0+e],c2);patch([0 0 1 1-e 0+e 0+e],[0 1 1 1-e 1-e 0+e],c3);plot([0 1 1 0 0],[0 0 1 1 0]);disp('D')
  mux : Mux  Inputs=2
      mask Display: e = 0.06;c1 = [120 150 230]/255;c2 = ([120 150 230]+0)/383;c3 = ([120 150 230]+128)/383;patch([0 1 1 0],[0 0 1 1],c1);patch([0 1 1 1-e 1-e 0+e],[0 0 1 1-e 0+e 0+e],c2);patch([0 0 1 1-e 0+e 0+e],[0 1 1 1-e 1-e 0+e],c3);plot([0 1 1 0 0],[0 0 1 1 0]);disp('Mux')
  "pd{1,2}" : Outport
      mask Display: e = 0.06;c1 = [120 230 180]/255;c2 = ([120 230 180]+0)/(256+128);c3 = ([120 230 180]+128)/(256+128);patch([0 1 1 0],[0 0 1 1],c1);patch([0 1 1 1-e 1-e 0+e],[0 0 1 1-e 0+e 0+e],c2);patch([0 0 1 1-e 0+e 0+e],[0 1 1 1-e 1-e 0+e],c3);plot([0 1 1 0 0],[0 0 1 1 0]);
  wires:
  "p{1}"/1 -> Delay 1/1
  Delay 1/1 -> Delay 2/1, mux/1
  Delay 2/1 -> mux/2
  mux/1 -> "pd{1,2}"/1
